simulink model "two_pos_simulink"  (R2021a)
settings: Solver=FixedStepAuto  StartTime=0.0  StopTime=500  FixedStep=1  RelTol=1e-3
values from neighbouring files (symbols this model uses):
  delay = 10    [two_position_controller_config.m]
  Hist = 0.3    [two_position_controller_config.m]
  k = 11/input_amplitude    (= 12.2222222222)    [two_position_controller_config.m]
  system_offset = 25    [two_position_controller_config.m]
  T = 250    [two_position_controller_config.m]
  u_max = 1    [two_position_controller_config.m]
  u_min = 0    [two_position_controller_config.m]
settings Model: Creator=dawidexpompa2000  LastModifiedBy=dawidexpompa2000

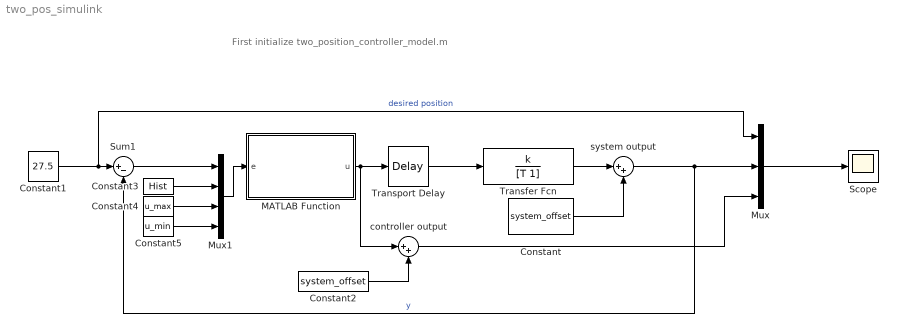
== system two_pos_simulink ==
  note: First initialize two_position_controller_model.m
  Constant : Constant  Value=system_offset
  Constant1 : Constant  Value=27.5
  Constant2 : Constant  Value=system_offset
  Constant3 : Constant  Value=Hist
  Constant4 : Constant  Value=u_max
  Constant5 : Constant  Value=u_min
  MATLAB Function : MATLAB Function  TreatAsAtomicUnit=on
  Mux : Mux  Inputs=3
  Mux1 : Mux
  Scope : Scope
  Sum1 : Sum  Inputs=|+-
  Transfer Fcn : TransferFcn  Numerator=k  Denominator=[T 1]
  Transport Delay : TransportDelay  DelayTime=delay
  controller output : Sum  Inputs=|++
  system output : Sum  Inputs=|++
  wires:
  Transport Delay/1 -> Transfer Fcn/1
  Transfer Fcn/1 -> system output/1
  Constant/1 -> system output/2
  system output/1 -> Sum1/2, Mux/2  "y"
  Mux/1 -> Scope/1
  Constant1/1 -> Mux/1, Sum1/1  "desired position"
  MATLAB Function/1(u) -> Transport Delay/1, controller output/1
  controller output/1 -> Mux/3
  Constant2/1 -> controller output/2
  Sum1/1 -> Mux1/1
  Mux1/1 -> MATLAB Function/1(e)
  Constant3/1 -> Mux1/2
  Constant4/1 -> Mux1/3
  Constant5/1 -> Mux1/4

== matlab function two_pos_simulink/MATLAB Function ==
  settings: updateMethod=DISCRETE
  data: e input; u output
function u = controller_two_position(e)

error = e(1);
H = e(2);
u_max = e(3);
u_min = e(4);

%static value
persistent u_value;
if isempty(u_value)
    u_value = 0;
end

%controller equation
if(error >= H/2) u_value=u_max; end
if(error < -H/2) u_value = u_min; end

u = u_value;
